simulink model "question1"  (Simulink 8.8)
settings: Solver=ode113  StartTime=0.0  StopTime=10.0  RelTol=1e-3
libraries: fuzblock x1, simulink x1
settings Model: Creator=Dreamer  LastModifiedBy=Dreamer
settings DataIOCC: LimitDataPoints=off  SaveFormat=Dataset  SignalLoggingSaveFormat=Dataset
settings OptimizationCC: LifeSpan=auto
settings DebuggingCC: UnderspecifiedInitializationDetection=Simplified  MergeDetectMultiDrivingBlocksExec=error  FcnCallInpInsideContextMsg=error  StateNameClashWarn=none  SFUnexpectedBacktrackingDiag=error  SFNoUnconditionalDefaultTransitionDiag=error  SFExecutionAtInitializationDiag=warning
settings HardwareCC: ProdBitPerPointer=64  ProdBitPerSizeT=64  ProdBitPerPtrDiffT=64  ProdLargestAtomicFloat=Float  ProdIntDivRoundTo=Zero  ProdEndianess=LittleEndian  ProdWordSize=64  ProdHWDeviceType=Intel->x86-64 (Windows64)
settings ModelReferenceCC: PropagateSignalLabelsOutOfModel=on
settings GRTTargetCC: TargetLangStandard=C99 (ISO)  GeneratePreprocessorConditionals=Use local settings  CombineOutputUpdateFcns=on  GRTInterface=off
settings ConfigComp: CovMetricSettings=dwe  CovHtmlReporting=off  CovSaveCumulativeToWorkspaceVar=off  CovSaveSingleToWorkspaceVar=off  CovExternalEMLEnable=on

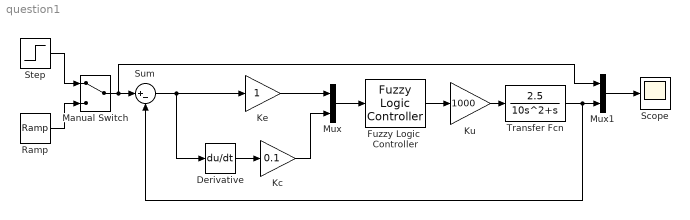
== system question1 ==
  Derivative : Derivative
  Fuzzy Logic  Controller : fuzblock/Fuzzy Logic  Controller  fis='question1.fis'
  Kc : Gain  Gain=0.1
  Ke : Gain
  Ku : Gain  Gain=1000
  Manual Switch : ManualSwitch
  Mux : Mux  Inputs=2
  Mux1 : Mux  Inputs=2
  Ramp : simulink/Sources/Ramp  slope=1  start=0  X0=0
  Scope : Scope
  Step : Step  SampleTime=0
  Sum : Sum  Inputs=|+-
  Transfer Fcn : TransferFcn  Numerator=[2.5]  Denominator=[10 1 0]
  wires:
  Fuzzy Logic  Controller/1 -> Ku/1
  Ku/1 -> Transfer Fcn/1
  Mux/1 -> Fuzzy Logic  Controller/1
  Ke/1 -> Mux/1
  Sum/1 -> Derivative/1, Ke/1
  Mux1/1 -> Scope/1
  Transfer Fcn/1 -> Sum/2, Mux1/2
  Derivative/1 -> Kc/1
  Kc/1 -> Mux/2
  Manual Switch/1 -> Mux1/1, Sum/1
  Step/1 -> Manual Switch/1
  Ramp/1 -> Manual Switch/2
